simulink model "radar2jammerr"  (R2024a)
settings: Solver=VariableStepAuto  StartTime=0.0  StopTime=inf  RelTol=1e-3
libraries: robotlib x6
settings Model: PacingRate=0.890000  Creator=bitdol  LastModifiedBy=bitdol

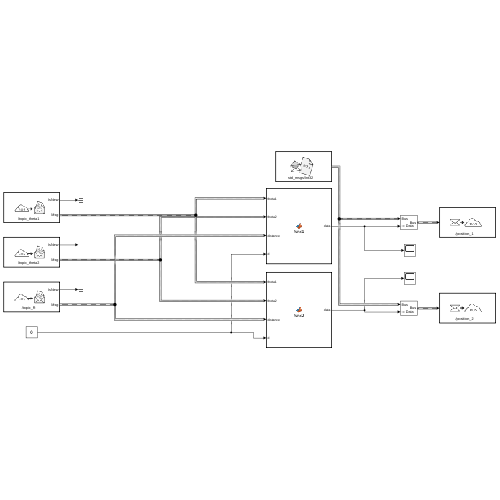
[thumbnail: Simulink's stored preview of the top-level diagram]
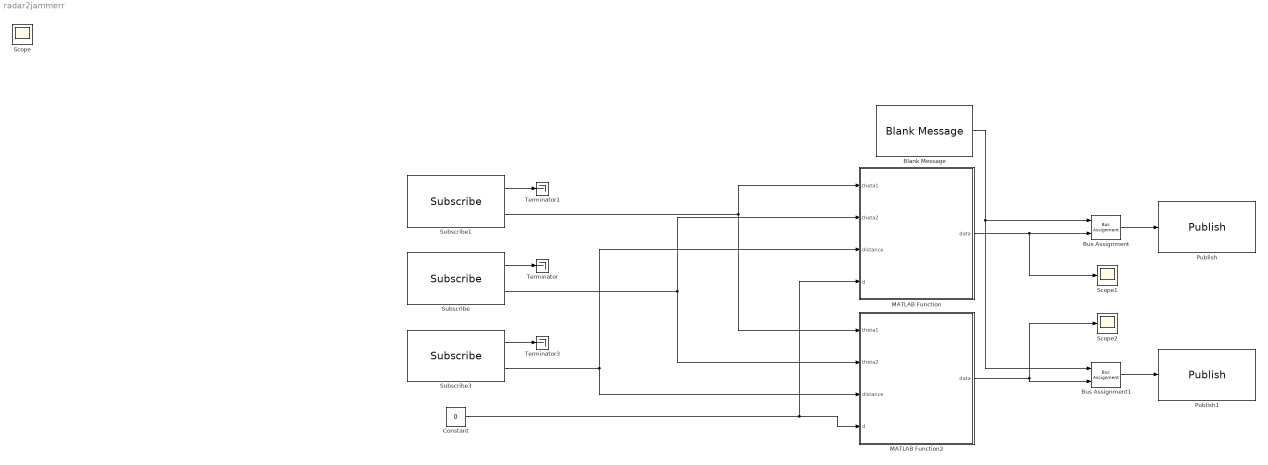
== system radar2jammerr ==
  Blank Message : robotlib/Blank Message  messageClass=Message  entityType=std_msgs/Int32  messageType=std_msgs/Int32  SampleTime=inf  legacyBusStruct=off
  Bus Assignment : BusAssignment  AssignedSignals=Data
  Bus Assignment1 : BusAssignment  AssignedSignals=Data
  Constant : Constant  Value=0
  MATLAB Function : MATLAB Function  TreatAsAtomicUnit=on
  MATLAB Function2 : MATLAB Function  TreatAsAtomicUnit=on
  Publish : robotlib/Publish  topicSource=Select from ROS network  topic=/position_1  messageType=std_msgs/Int32  legacyBusStruct=off  messageQueueLength=1
  Publish1 : robotlib/Publish  topicSource=Select from ROS network  topic=/position_2  messageType=std_msgs/Int32  legacyBusStruct=off  messageQueueLength=1
  Scope1 : Scope
  Scope2 : Scope
  Subscribe : robotlib/Subscribe  topicSource=Select from ROS network  topic=/topic_theta2  messageType=std_msgs/Int32  SampleTime=-1  legacyBusStruct=off  messageQueueLength=1
  Subscribe1 : robotlib/Subscribe  topicSource=Select from ROS network  topic=/topic_theta1  messageType=std_msgs/Int32  SampleTime=-1  legacyBusStruct=off  messageQueueLength=1
  Subscribe3 : robotlib/Subscribe  topicSource=Select from ROS network  topic=/topic_R  messageType=std_msgs/Int32  SampleTime=-1  legacyBusStruct=off  messageQueueLength=1
  Terminator : Terminator
  Terminator1 : Terminator
  Terminator3 : Terminator
  Scope : Scope
  wires:
  Subscribe3/1 -> Terminator3/1
  Subscribe1/1 -> Terminator1/1
  Bus Assignment1/1 -> Publish1/1
  MATLAB Function2/1(data) -> Bus Assignment1/2, Scope2/1
  Subscribe/1 -> Terminator/1
  Subscribe/2 -> MATLAB Function2/2(theta2), MATLAB Function/2(theta2)
  MATLAB Function/1(data) -> Scope1/1, Bus Assignment/2
  Constant/1 -> MATLAB Function2/4(d), MATLAB Function/4(d)
  Bus Assignment/1 -> Publish/1
  Blank Message/1 -> Bus Assignment1/1, Bus Assignment/1
  Subscribe1/2 -> MATLAB Function2/1(theta1), MATLAB Function/1(theta1)
  Subscribe3/2 -> MATLAB Function2/3(distance), MATLAB Function/3(distance)

== matlab function radar2jammerr/MATLAB Function ==
  data: theta1 input; theta2 input; distance input; data output; d input
function data = func1(theta1, theta2, distance, d)
    a1 = double((theta1.Data - 1024) * (180 / 2048));
    a2 = double((theta2.Data) * (180 / 2048));
    r = double(distance.Data);
    x = r * cosd(a2) * cosd(a1);
    y = r * cosd(a2) * sind(a1);
    output1 = abs(atan2d(y, (x - d)));

    data = int32((output1) * (2048 / 180) + 1024);

== matlab function radar2jammerr/MATLAB Function2 ==
  data: theta1 input; theta2 input; distance input; data output; d input
function data = func2(theta1, theta2, distance, d)
    a1 = double((theta1.Data - 1024) * (180 / 2048));
    a2 = double((theta2.Data ) * (180 / 2048));
    r = double(distance.Data);

    x = r * cosd(a2) * cosd(a1);
    y = r * cosd(a2) * sind(a1);
    z = r * sind(a2);

    output2 = abs(atan2d(z , sqrt((x - d)^2 + y^2)));

    data = int32(output2*2048/180);
end
